simulink library "DAQ_lib_HallPositionTorque"  (R2014b)
settings: Solver=ode45  StartTime=0.0  StopTime=10.0  RelTol=1e-3
undefined symbols (not defined in the file): A_lpf_velocity, ANOMALY_INIT, B1_lpf_velocity, B2_lpf_velocity, Calibration, EnableFT, EncoderAngleLimits, EncoderFiltSys, EncoderThreshold, FTCalibration, GearOffsets, IMUAngleLimits, IMUCommand, IMUThreshold, IMUTorsoOffsets, m_XR17D15x, MAX_ANOMALY, MedullaCommand, MicrostrainFiltSys, MODBUS_TIMEOUT, ResetDAQ, ResetYaw, sample_time, standard, STREAMING_TIMEOUT, TareFT, TorsoCOMOffsets, Ts, TsCAN, TsKVH, UseMicrostrainRate
libraries: xpcethercatlib x207, simulink x53, canmsglib x21, speedgoatlib x13, slrtlib x5, speedgoatlib_IO601 x5, dspswit3 x2, dspmtrx3 x2, xpcseriallib x1, SpeedgoatModified x1
(part 1 of 7)
settings Model: Creator=rosshart  LastModifiedBy=rosshart

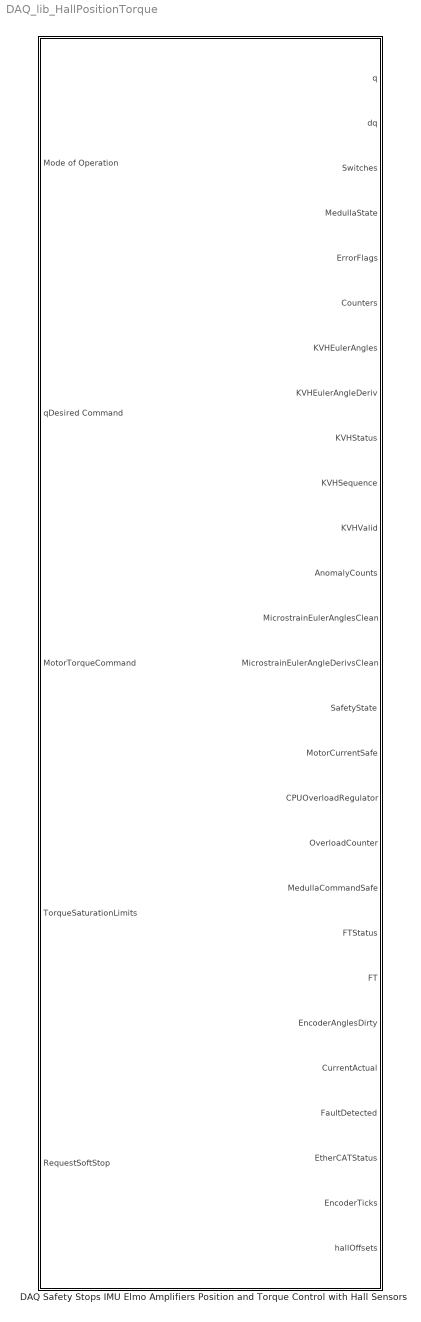
== system DAQ_lib_HallPositionTorque ==
  DAQ Safety Stops IMU Elmo Amplifiers Position and Torque Control with Hall Sensors : Subsystem  AncestorBlock=|
      | DAQ_lib/DAQ
      | Safety Stops
      | IMU
      | Elmo Amplifiers
      | Position and Torque Control with Hall Sensors

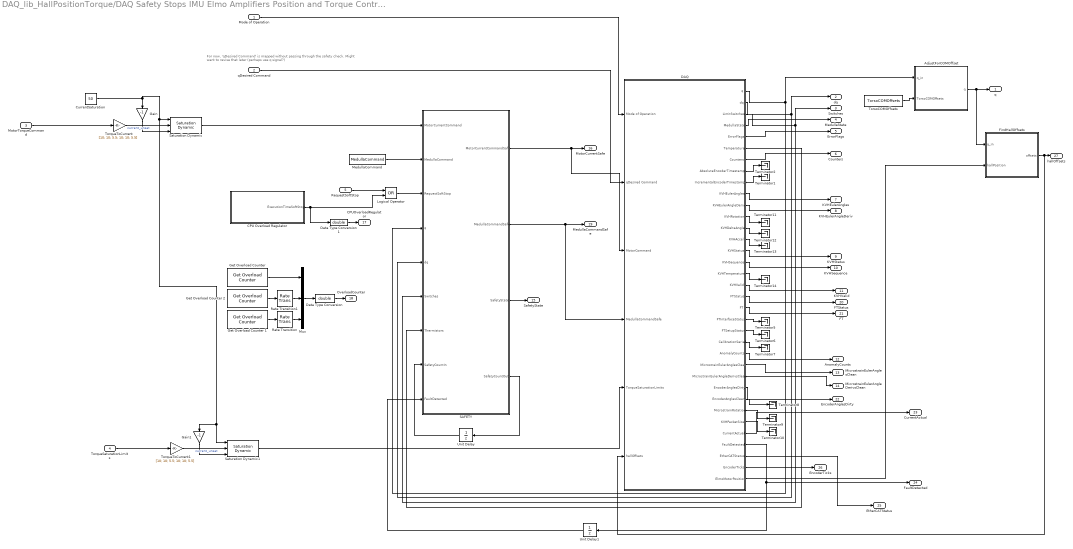
== system DAQ_lib_HallPositionTorque/DAQ Safety Stops IMU Elmo Amplifiers Position and Torque Control with Hall Sensors ==
  note: For now, 'qDesired Command' is mapped without passing through the safety check.
      | Might want to revise that later (perhaps use q signal?)
  Mode of Operation : Inport
  qDesired Command : Inport  Port=2
  MotorTorqueCommand : Inport  Port=3
  TorqueSaturationLimits : Inport  Port=4
  RequestSoftStop : Inport  Port=5
  AdjustForCOMOffset : MATLAB Function  TreatAsAtomicUnit=on
  CPU Overload Regulator : Subsystem
  CurrentSaturation : Constant  Value=50
  DAQ : Subsystem
  Data Type Conversion : DataTypeConversion  OutDataTypeStr=double
  Data Type Conversion1 : DataTypeConversion  OutDataTypeStr=double
  FindHallOffsets : MATLAB Function  TreatAsAtomicUnit=on
  Gain : Gain  Gain=-1
  Gain1 : Gain  Gain=-1
  "Get Overload Counter " : slrtlib/Target Management/Execution Parameters/Get Overload Counter   ts=Ts
  Get Overload Counter 1 : slrtlib/Target Management/Execution Parameters/Get Overload Counter   ts=TsMicrostrain
  Get Overload Counter 2 : slrtlib/Target Management/Execution Parameters/Get Overload Counter   ts=TsKVH
  Logical Operator : Logic  Operator=OR  OutDataTypeStr=boolean
  MedullaCommand : Constant  Value=MedullaCommand
  Mux : Mux  Inputs=3
  Rate Transition : RateTransition
  Rate Transition1 : RateTransition
  SAFETY : MATLAB Function  TreatAsAtomicUnit=on
  Saturation Dynamic : simulink/Discontinuities/Saturation Dynamic  OutMin=[]  OutMax=[]  OutDataTypeStr=Inherit: Same as second input  OutDataType=fixdt(1, 16)  OutScaling=2^-10  DoSatur=off
  Saturation Dynamic1 : simulink/Discontinuities/Saturation Dynamic  OutMin=[]  OutMax=[]  OutDataTypeStr=Inherit: Same as second input  OutDataType=fixdt(1, 16)  OutScaling=2^-10  DoSatur=off
  Terminator{1..2,5..14} (12 alike) : Terminator
  TorqueToCurrent : Gain  Gain=[10; 10; 5.5; 10; 10; 5.5]
  TorqueToCurrent1 : Gain  Gain=[10; 10; 5.5; 10; 10; 5.5]
  TorsoCOMOffsets : Constant  Value=TorsoCOMOffsets
  Unit Delay : UnitDelay  SampleTime=-1
  Unit Delay1 : UnitDelay  SampleTime=-1
  q : Outport
  dq : Outport  Port=2
  Switches : Outport  Port=3
  MedullaState : Outport  Port=4
  ErrorFlags : Outport  Port=5
  Counters : Outport  Port=6
  KVHEulerAngles : Outport  Port=7
  KVHEulerAngleDeriv : Outport  Port=8
  KVHStatus : Outport  Port=9
  KVHSequence : Outport  Port=10
  KVHValid : Outport  Port=11
  AnomalyCounts : Outport  Port=12
  MicrostrainEulerAnglesClean : Outport  Port=13
  MicrostrainEulerAngleDerivsClean : Outport  Port=14
  SafetyState : Outport  Port=15
  MotorCurrentSafe : Outport  Port=16
  CPUOverloadRegulator : Outport  Port=17
  OverloadCounter : Outport  Port=18
  MedullaCommandSafe : Outport  Port=19
  FTStatus : Outport  Port=20
  FT : Outport  Port=21
  EncoderAnglesDirty : Outport  Port=22
  CurrentActual : Outport  Port=23
  FaultDetected : Outport  Port=24
  EtherCATStatus : Outport  Port=25
  EncoderTicks : Outport  Port=26
  hallOffsets : Outport  Port=27
  wires:
  FindHallOffsets/1(offsets) -> hallOffsets/1, DAQ/6(hallOffsets)
  DAQ/35(ElmoMotorPosition) -> FindHallOffsets/2(hallPosition)
  TorqueSaturationLimits/1 -> TorqueToCurrent1/1
  TorqueToCurrent1/1 -> Saturation Dynamic1/2  "current_unsat"
  Gain1/1 -> Saturation Dynamic1/3
  Saturation Dynamic1/1 -> DAQ/5(TorqueSaturationLimits)
  DAQ/34(EncoderTicks) -> EncoderTicks/1
  DAQ/33(EtherCATStatus) -> EtherCATStatus/1
  MotorTorqueCommand/1 -> TorqueToCurrent/1
  DAQ/1(q) -> AdjustForCOMOffset/1(q_in), SAFETY/4(q)
  DAQ/2(dq) -> dq/1, SAFETY/5(dq)
  DAQ/3(LimitSwitches) -> Switches/1, SAFETY/6(Switches)
  SAFETY/3(SafetyState) -> SafetyState/1
  TorqueToCurrent/1 -> Saturation Dynamic/2  "current_unsat"
  DAQ/4(MedullaState) -> MedullaState/1
  DAQ/5(ErrorFlags) -> ErrorFlags/1
  Gain/1 -> Saturation Dynamic/3
  Saturation Dynamic/1 -> SAFETY/1(MotorCurrentCommand)
  SAFETY/2(MedullaCommandSafe) -> DAQ/4(MedullaCommandSafe), MedullaCommandSafe/1
  SAFETY/4(SafetyCountOut) -> Unit Delay/1
  Unit Delay/1 -> SAFETY/8(SafetyCountIn)
  DAQ/6(Temperature) -> SAFETY/7(Thermistors)
  DAQ/7(Counters) -> Counters/1
  AdjustForCOMOffset/1(q) -> q/1, FindHallOffsets/1(q_in)
  SAFETY/1(MotorCurrentCommandSafe) -> MotorCurrentSafe/1, DAQ/3(MotorCommand)
  DAQ/10(KVHEulerAngles) -> KVHEulerAngles/1
  DAQ/11(KVHEulerAngleDeriv) -> KVHEulerAngleDeriv/1
  DAQ/16(KVHSequence) -> KVHSequence/1
  DAQ/18(KVHValid) -> KVHValid/1
  DAQ/15(KVHStatus) -> KVHStatus/1
  DAQ/9(IncrementalEncoderTimestamps) -> Terminator1/1
  DAQ/24(AnomalyCounts) -> AnomalyCounts/1
  DAQ/8(AbsoluteEncoderTimestamps) -> Terminator2/1
  DAQ/25(MicrostrainEulerAnglesClean) -> MicrostrainEulerAnglesClean/1
  DAQ/26(MicrostrainEulerAngleDerivsClean) -> MicrostrainEulerAngleDerivsClean/1
  Logical Operator/1 -> SAFETY/3(RequestSoftStop)
  RequestSoftStop/1 -> Logical Operator/1
  CPU Overload Regulator/1(ExecutionTimeSoftStop) -> Logical Operator/2, Data Type Conversion1/1
  Data Type Conversion1/1 -> CPUOverloadRegulator/1
  MedullaCommand/1 -> SAFETY/2(MedullaCommand)
  CurrentSaturation/1 -> Gain/1, Saturation Dynamic/1, Saturation Dynamic1/1, Gain1/1
  TorsoCOMOffsets/1 -> AdjustForCOMOffset/2(TorsoCOMOffsets)
  DAQ/28(EncoderAnglesClean) -> Terminator8/1
  DAQ/29(MicrostrainRotation) -> Terminator9/1
  DAQ/30(KVHPacketSize) -> Terminator10/1
  DAQ/19(FTStatus) -> FTStatus/1
  DAQ/20(FT) -> FT/1
  DAQ/21(FTInterfaceStatus) -> Terminator5/1
  DAQ/23(CalibrationSerial) -> Terminator7/1
  DAQ/22(FTSetupStatus) -> Terminator6/1
  DAQ/14(KVHAccel) -> Terminator13/1
  DAQ/13(KVHDeltaAngle) -> Terminator12/1
  DAQ/12(KVHRotation) -> Terminator11/1
  DAQ/17(KVHTemperature) -> Terminator14/1
  "Get Overload Counter "/1 -> Mux/1
  Data Type Conversion/1 -> OverloadCounter/1
  Get Overload Counter 1/1 -> Rate Transition/1
  Mux/1 -> Data Type Conversion/1
  Rate Transition/1 -> Mux/3
  Get Overload Counter 2/1 -> Rate Transition1/1
  Rate Transition1/1 -> Mux/2
  DAQ/27(EncoderAnglesDirty) -> EncoderAnglesDirty/1
  DAQ/31(CurrentActual) -> CurrentActual/1
  DAQ/32(FaultDetected) -> Unit Delay1/1, FaultDetected/1
  Unit Delay1/1 -> SAFETY/9(FaultDetected)
  qDesired Command/1 -> DAQ/2(qDesired Command)
  Mode of Operation/1 -> DAQ/1(Mode of Operation)

== system DAQ_lib_HallPositionTorque/DAQ Safety Stops IMU Elmo Amplifiers Position and Torque Control with Hall Sensors/CPU Overload Regulator ==
  Bias : Bias  Bias=-1
  Compare To Constant : simulink/Logic and Bit Operations/Compare To Constant  relop=>=  const=Ts  OutDataTypeStr=boolean
  Compare To Constant1 : simulink/Logic and Bit Operations/Compare To Constant  relop=>=  const=Ts*10  OutDataTypeStr=boolean
  Compare To Zero : simulink/Logic and Bit Operations/Compare To Zero  relop===  OutDataTypeStr=boolean
  Reset CPU Overload Count : Subsystem  TreatAsAtomicUnit=on
  ResetExecutionDelaySteps : Constant  Value=50  SampleTime=Ts
  Resettable Delay : Delay  DelayLength=1  InitialConditionSource=Input port  ExternalReset=Level hold
      settings: InputPortMap=u0,r5,p4
  "Task Execution Time " : slrtlib/Target Management/Execution Parameters/Task Execution Time   ts=Ts
  ExecutionTimeSoftStop : Outport
  wires:
  Compare To Constant/1 -> Resettable Delay/2
  ResetExecutionDelaySteps/1 -> Resettable Delay/3
  "Task Execution Time "/1 -> Compare To Constant1/1, Compare To Constant/1
  Compare To Zero/1 -> Reset CPU Overload Count/Enable
  Compare To Constant1/1 -> ExecutionTimeSoftStop/1  "Request Soft Stop"
  Resettable Delay/1 -> Compare To Zero/1, Bias/1
  Bias/1 -> Resettable Delay/1

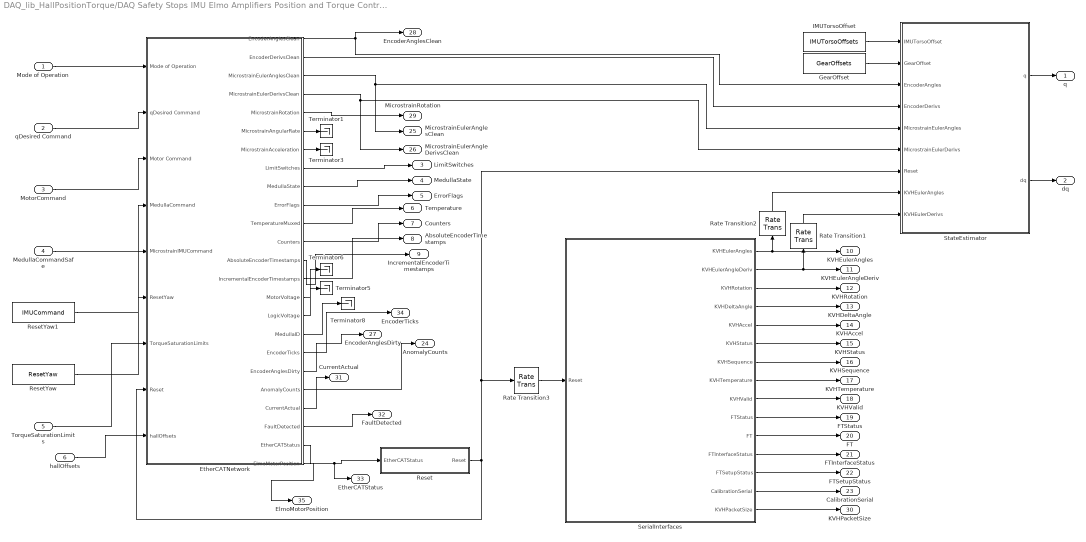
== system DAQ_lib_HallPositionTorque/DAQ Safety Stops IMU Elmo Amplifiers Position and Torque Control with Hall Sensors/DAQ ==
  Mode of Operation : Inport
  qDesired Command : Inport  Port=2
  MotorCommand : Inport  Port=3
  MedullaCommandSafe : Inport  Port=4
  TorqueSaturationLimits : Inport  Port=5
  hallOffsets : Inport  Port=6
  EtherCATNetwork : Subsystem
  GearOffset : Constant  Value=GearOffsets
  IMUTorsoOffset : Constant  Value=IMUTorsoOffsets
  Rate Transition1 : RateTransition  OutPortSampleTime=Ts
  Rate Transition2 : RateTransition  OutPortSampleTime=Ts
  Rate Transition3 : RateTransition  OutPortSampleTime=0.001
  Reset : Subsystem
  ResetYaw : Constant  Value=ResetYaw  OutDataTypeStr=boolean
  ResetYaw1 : Constant  Value=IMUCommand
  SerialInterfaces : Subsystem  TreatAsAtomicUnit=on  SystemSampleTime=TsKVH
  StateEstimator : Subsystem
  Terminator{1,3,5..6,8} (5 alike) : Terminator
  q : Outport
  dq : Outport  Port=2
  LimitSwitches : Outport  Port=3
  MedullaState : Outport  Port=4
  ErrorFlags : Outport  Port=5
  Temperature : Outport  Port=6
  Counters : Outport  Port=7
  AbsoluteEncoderTimestamps : Outport  Port=8
  IncrementalEncoderTimestamps : Outport  Port=9
  KVHEulerAngles : Outport  Port=10
  KVHEulerAngleDeriv : Outport  Port=11
  KVHRotation : Outport  Port=12
  KVHDeltaAngle : Outport  Port=13
  KVHAccel : Outport  Port=14
  KVHStatus : Outport  Port=15
  KVHSequence : Outport  Port=16
  KVHTemperature : Outport  Port=17
  KVHValid : Outport  Port=18
  FTStatus : Outport  Port=19
  FT : Outport  Port=20
  FTInterfaceStatus : Outport  Port=21
  FTSetupStatus : Outport  Port=22
  CalibrationSerial : Outport  Port=23
  AnomalyCounts : Outport  Port=24
  MicrostrainEulerAnglesClean : Outport  Port=25
  MicrostrainEulerAngleDerivsClean : Outport  Port=26
  EncoderAnglesDirty : Outport  Port=27
  EncoderAnglesClean : Outport  Port=28
  MicrostrainRotation : Outport  Port=29
  KVHPacketSize : Outport  Port=30
  CurrentActual : Outport  Port=31
  FaultDetected : Outport  Port=32
  EtherCATStatus : Outport  Port=33
  EncoderTicks : Outport  Port=34
  ElmoMotorPosition : Outport  Port=35
  wires:
  hallOffsets/1 -> EtherCATNetwork/9(hallOffsets)
  EtherCATNetwork/24(ElmoMotorPosition) -> ElmoMotorPosition/1
  TorqueSaturationLimits/1 -> EtherCATNetwork/7(TorqueSaturationLimits)
  ResetYaw/1 -> EtherCATNetwork/6(ResetYaw)
  Rate Transition3/1 -> SerialInterfaces/1(Reset)
  EtherCATNetwork/19(EncoderAnglesDirty) -> EncoderAnglesDirty/1
  SerialInterfaces/15(KVHPacketSize) -> KVHPacketSize/1
  EtherCATNetwork/6(MicrostrainAngularRate) -> Terminator1/1
  EtherCATNetwork/2(EncoderDerivsClean) -> StateEstimator/4(EncoderDerivs)
  Rate Transition1/1 -> StateEstimator/9(KVHEulerDerivs)
  EtherCATNetwork/10(ErrorFlags) -> ErrorFlags/1
  EtherCATNetwork/8(LimitSwitches) -> LimitSwitches/1
  EtherCATNetwork/5(MicrostrainRotation) -> MicrostrainRotation/1
  EtherCATNetwork/15(MotorVoltage) -> Terminator6/1
  EtherCATNetwork/14(IncrementalEncoderTimestamps) -> IncrementalEncoderTimestamps/1
  EtherCATNetwork/16(LogicVoltage) -> Terminator5/1
  EtherCATNetwork/17(MedullaID) -> Terminator8/1
  SerialInterfaces/3(KVHRotation) -> KVHRotation/1
  SerialInterfaces/1(KVHEulerAngles) -> KVHEulerAngles/1, Rate Transition2/1
  MotorCommand/1 -> EtherCATNetwork/3(Motor Command)
  SerialInterfaces/11(FT) -> FT/1
  StateEstimator/1(q) -> q/1
  IMUTorsoOffset/1 -> StateEstimator/1(IMUTorsoOffset)
  SerialInterfaces/13(FTSetupStatus) -> FTSetupStatus/1
  EtherCATNetwork/20(AnomalyCounts) -> AnomalyCounts/1
  EtherCATNetwork/12(Counters) -> Counters/1
  EtherCATNetwork/9(MedullaState) -> MedullaState/1
  StateEstimator/2(dq) -> dq/1
  EtherCATNetwork/13(AbsoluteEncoderTimestamps) -> AbsoluteEncoderTimestamps/1
  SerialInterfaces/10(FTStatus) -> FTStatus/1
  SerialInterfaces/12(FTInterfaceStatus) -> FTInterfaceStatus/1
  SerialInterfaces/2(KVHEulerAngleDeriv) -> KVHEulerAngleDeriv/1, Rate Transition1/1
  SerialInterfaces/8(KVHTemperature) -> KVHTemperature/1
  EtherCATNetwork/11(TemperatureMuxed) -> Temperature/1
  EtherCATNetwork/7(MicrostrainAcceleration) -> Terminator3/1
  EtherCATNetwork/18(EncoderTicks) -> EncoderTicks/1
  SerialInterfaces/14(CalibrationSerial) -> CalibrationSerial/1
  SerialInterfaces/5(KVHAccel) -> KVHAccel/1
  SerialInterfaces/7(KVHSequence) -> KVHSequence/1
  SerialInterfaces/9(KVHValid) -> KVHValid/1
  SerialInterfaces/6(KVHStatus) -> KVHStatus/1
  SerialInterfaces/4(KVHDeltaAngle) -> KVHDeltaAngle/1
  GearOffset/1 -> StateEstimator/2(GearOffset)
  EtherCATNetwork/3(MicrostrainEulerAnglesClean) -> MicrostrainEulerAnglesClean/1, StateEstimator/5(MicrostrainEulerAngles)
  EtherCATNetwork/4(MicrostrainEulerDerivsClean) -> StateEstimator/6(" MicrostrainEulerDerivs"), MicrostrainEulerAngleDerivsClean/1
  Reset/1(Reset) -> StateEstimator/7(Reset), Rate Transition3/1, EtherCATNetwork/8(Reset)
  Rate Transition2/1 -> StateEstimator/8(KVHEulerAngles)
  EtherCATNetwork/1(EncoderAnglesClean) -> EncoderAnglesClean/1, StateEstimator/3(EncoderAngles)
  MedullaCommandSafe/1 -> EtherCATNetwork/4(MedullaCommand)
  ResetYaw1/1 -> EtherCATNetwork/5(MicrostrainIMUCommand)
  EtherCATNetwork/21(CurrentActual) -> CurrentActual/1
  EtherCATNetwork/22(FaultDetected) -> FaultDetected/1
  qDesired Command/1 -> EtherCATNetwork/2(qDesired Command)
  EtherCATNetwork/23(EtherCATStatus) -> EtherCATStatus/1, Reset/1(EtherCATStatus)
  Mode of Operation/1 -> EtherCATNetwork/1(Mode of Operation)

== system DAQ_lib_HallPositionTorque/DAQ Safety Stops IMU Elmo Amplifiers Position and Torque Control with Hall Sensors/CPU Overload Regulator/Reset CPU Overload Count ==
  Enable : EnablePort
  Constant1 : Constant  Value=0
  Set Overload Counter 1 : slrtlib/Target Management/Execution Parameters/Set Overload Counter   ts=-1
  wires:
  Constant1/1 -> Set Overload Counter 1/1

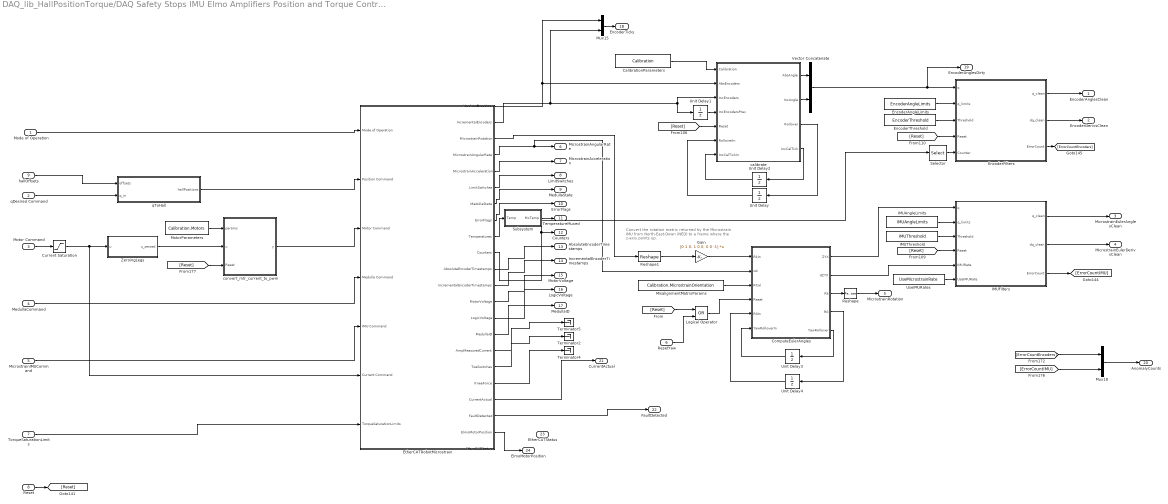
== system DAQ_lib_HallPositionTorque/DAQ Safety Stops IMU Elmo Amplifiers Position and Torque Control with Hall Sensors/DAQ/EtherCATNetwork ==
  note: Convert the rotation matrix returned by the
      | Microstrain IMU from North-East-Down
      | (NED) to a frame where the z-axis points up.
  Mode of Operation : Inport
  qDesired Command : Inport  Port=2
  Motor Command : Inport  Port=3
  MedullaCommand : Inport  Port=4
  MicrostrainIMUCommand : Inport  Port=5
  ResetYaw : Inport  Port=6
  TorqueSaturationLimits : Inport  Port=7
  Reset : Inport  Port=8
  hallOffsets : Inport  Port=9
  CalibrationParameters : Constant  Value=Calibration  OutDataTypeStr=Bus: RobotCalibrationBus
  ComputeEulerAngles : MATLAB Function  TreatAsAtomicUnit=on
  Current Saturation : Saturate  UpperLimit=50  LowerLimit=-50
  EncoderAngleLimits : Constant  Value=EncoderAngleLimits
  EncoderFilters : Subsystem  TreatAsAtomicUnit=on
  EncoderThreshold : Constant  Value=EncoderThreshold
  EtherCATRobotMicrostrain : Subsystem
  Gain : Gain  Gain=[0 1 0; 1 0 0; 0 0 -1]  Multiplication=Matrix(K*u)
  IMUAngleLimits : Constant  Value=IMUAngleLimits
  IMUFilters : Subsystem  TreatAsAtomicUnit=on
  IMUThreshold : Constant  Value=IMUThreshold
  Logical Operator : Logic  Operator=OR  OutDataTypeStr=boolean
  MisalignmentMatrixParams : Constant  Value=Calibration.MicrostrainOrientation
  MotorParameters : Constant  Value=Calibration.Motors
  Mux15 : Mux  Inputs=2
  Mux18 : Mux  Inputs=2
  Reshape : Reshape
  Reshape1 : Reshape  OutputDimensionality=Customize  OutputDimensions=[3,3]
  Selector : Selector  IndexMode=Zero-based  InputPortWidth=7  Indices=[0 1 3 4 0 1 3 4 2 5 0 1 3 4 2 5 6 6 6]
  Subsystem : Subsystem
  Terminator2 : Terminator
  Terminator4 : Terminator
  Terminator5 : Terminator
  Unit Delay : UnitDelay  InitialCondition=zeros(9,1)  SampleTime=-1
  Unit Delay1 : UnitDelay  SampleTime=-1
  Unit Delay2 : UnitDelay  InitialCondition=zeros(6,1)  SampleTime=-1
  Unit Delay3 : UnitDelay  InitialCondition=[0; 0]  SampleTime=-1
  Unit Delay4 : UnitDelay  InitialCondition=zeros(3,3)  SampleTime=-1
  UseIMURates : Constant  Value=UseMicrostrainRate
  Vector Concatenate : Concatenate
  ZeroingLegs : MATLAB Function  TreatAsAtomicUnit=on
  calibrate : MATLAB Function  TreatAsAtomicUnit=on
  convert_mtr_current_to_pwm : MATLAB Function  TreatAsAtomicUnit=on
  qToHall : MATLAB Function  TreatAsAtomicUnit=on
  EncoderAnglesClean : Outport
  EncoderDerivsClean : Outport  Port=2
  MicrostrainEulerAnglesClean : Outport  Port=3
  MicrostrainEulerDerivsClean : Outport  Port=4
  MicrostrainRotation : Outport  Port=5
  MicrostrainAngularRate : Outport  Port=6
  MicrostrainAcceleration : Outport  Port=7
  LimitSwitches : Outport  Port=8
  MedullaState : Outport  Port=9
  ErrorFlags : Outport  Port=10
  TemperatureMuxed : Outport  Port=11
  Counters : Outport  Port=12
  AbsoluteEncoderTimestamps : Outport  Port=13
  IncrementalEncoderTimestamps : Outport  Port=14
  MotorVoltage : Outport  Port=15
  LogicVoltage : Outport  Port=16
  MedullaID : Outport  Port=17
  EncoderTicks : Outport  Port=18
  EncoderAnglesDirty : Outport  Port=19
  AnomalyCounts : Outport  Port=20
  CurrentActual : Outport  Port=21
  FaultDetected : Outport  Port=22
  EtherCATStatus : Outport  Port=23
  ElmoMotorPosition : Outport  Port=24
  wires:
  hallOffsets/1 -> qToHall/1(offsets)
  EtherCATRobotMicrostrain/21(ElmoMotorPosition) -> ElmoMotorPosition/1
  ? -> EtherCATStatus/1
  TorqueSaturationLimits/1 -> EtherCATRobotMicrostrain/7(TorqueSaturationLimits)
  EtherCATRobotMicrostrain/17(ToeSwitches) -> Terminator2/1
  EtherCATRobotMicrostrain/16(AmpMeasuredCurrent) -> Terminator5/1
  MicrostrainIMUCommand/1 -> EtherCATRobotMicrostrain/5(IMU Command)
  MedullaCommand/1 -> EtherCATRobotMicrostrain/4(Medulla Command)
  CalibrationParameters/1 -> calibrate/1(Calibration)
  calibrate/3(Rollover) -> Unit Delay/1
  Unit Delay/1 -> calibrate/6(RolloverIn)
  [Reset] -> calibrate/5(Reset)
  Unit Delay1/1 -> calibrate/4(IncEncodersPrev)
  Unit Delay2/1 -> calibrate/7(IncCalTickIn)
  calibrate/4(IncCalTick) -> Unit Delay2/1
  [Reset] -> convert_mtr_current_to_pwm/3(Reset)
  Motor Command/1 -> Current Saturation/1
  MotorParameters/1 -> convert_mtr_current_to_pwm/1(params)
  Current Saturation/1 -> EtherCATRobotMicrostrain/6(Current Command), ZeroingLegs/1(u)
  convert_mtr_current_to_pwm/1(y) -> EtherCATRobotMicrostrain/3(Motor Command)
  Mux15/1 -> EncoderTicks/1
  EtherCATRobotMicrostrain/18(KneeForce) -> Terminator4/1
  EtherCATRobotMicrostrain/7(MedullaState) -> MedullaState/1
  Subsystem/1(MxTemp) -> TemperatureMuxed/1
  EtherCATRobotMicrostrain/9(Temperatures) -> Subsystem/1(Temp)
  EtherCATRobotMicrostrain/8(ErrorFlags) -> ErrorFlags/1
  EtherCATRobotMicrostrain/6(LimitSwitches) -> LimitSwitches/1
  EtherCATRobotMicrostrain/13(MotorVoltage) -> MotorVoltage/1
  EtherCATRobotMicrostrain/14(LogicVoltage) -> LogicVoltage/1
  EtherCATRobotMicrostrain/5(MicrostrainAcceleration) -> MicrostrainAcceleration/1
  EtherCATRobotMicrostrain/11(AbsoluteEncoderTimestamps) -> AbsoluteEncoderTimestamps/1
  EtherCATRobotMicrostrain/12(IncrementalEncoderTimestamps) -> IncrementalEncoderTimestamps/1
  EtherCATRobotMicrostrain/15(MedullaID) -> MedullaID/1
  EtherCATRobotMicrostrain/1(AbsoluteEncoders) -> Mux15/1, calibrate/2(AbsEncoders)
  EtherCATRobotMicrostrain/2(IncrementalEncoders) -> Mux15/2, calibrate/3(IncEncoders), Unit Delay1/1
  ComputeEulerAngles/1(ZYX) -> IMUFilters/1(q)
  [Reset] -> IMUFilters/4(Reset)
  IMUFilters/3(ErrorCount) -> [ErrorCountIMU]
  IMUThreshold/1 -> IMUFilters/3(Threshold)
  EtherCATRobotMicrostrain/10(Counters) -> Counters/1, Selector/1
  IMUAngleLimits/1 -> IMUFilters/2(q_limits)
  Selector/1 -> EncoderFilters/5(Counter)
  UseIMURates/1 -> IMUFilters/6(UseIMURate)
  EncoderFilters/3(ErrorCount) -> [ErrorCountEncoders]
  IMUFilters/2(dq_clean) -> MicrostrainEulerDerivsClean/1
  [Reset] -> EncoderFilters/4(Reset)
  EncoderAngleLimits/1 -> EncoderFilters/2(q_limits)
  EncoderFilters/1(q_clean) -> EncoderAnglesClean/1
  IMUFilters/1(q_clean) -> MicrostrainEulerAnglesClean/1
  EncoderFilters/2(dq_clean) -> EncoderDerivsClean/1
  EncoderThreshold/1 -> EncoderFilters/3(Threshold)
  calibrate/1(AbsAngle) -> Vector Concatenate/1
  calibrate/2(IncAngle) -> Vector Concatenate/2
  Vector Concatenate/1 -> EncoderAnglesDirty/1, EncoderFilters/1(q)
  ComputeEulerAngles/2(dZYX) -> IMUFilters/5(IMURate)
  Mux18/1 -> AnomalyCounts/1
  [ErrorCountEncoders] -> Mux18/1
  [ErrorCountIMU] -> Mux18/2
  MisalignmentMatrixParams/1 -> ComputeEulerAngles/3(RCal)
  Unit Delay4/1 -> ComputeEulerAngles/5(R0In)
  ComputeEulerAngles/4(R0) -> Unit Delay4/1
  ComputeEulerAngles/3(Rk) -> Reshape/1
  [Reset] -> Logical Operator/1
  Reshape/1 -> MicrostrainRotation/1
  EtherCATRobotMicrostrain/3(MicrostrainRotation) -> Reshape1/1
  EtherCATRobotMicrostrain/4(MicrostrainAngularRate) -> MicrostrainAngularRate/1, ComputeEulerAngles/2(wk)
  ComputeEulerAngles/5(YawRollover) -> Unit Delay3/1
  Unit Delay3/1 -> ComputeEulerAngles/6(YawRolloverIn)
  ResetYaw/1 -> Logical Operator/2
  Logical Operator/1 -> ComputeEulerAngles/4(Reset)
  Reshape1/1 -> Gain/1
  Gain/1 -> ComputeEulerAngles/1(RkIn)
  Reset/1 -> [Reset]
  EtherCATRobotMicrostrain/19(CurrentActual) -> CurrentActual/1
  EtherCATRobotMicrostrain/20(FaultDetected) -> FaultDetected/1
  ZeroingLegs/1(u_zeroed) -> convert_mtr_current_to_pwm/2(u)
  qDesired Command/1 -> qToHall/2(q_in)
  Mode of Operation/1 -> EtherCATRobotMicrostrain/1(Mode of Operation)
  qToHall/1(hallPositions) -> EtherCATRobotMicrostrain/2(Position Command)

== system DAQ_lib_HallPositionTorque/DAQ Safety Stops IMU Elmo Amplifiers Position and Torque Control with Hall Sensors/DAQ/Reset ==
  note: EtherCATStatus is a vector of six elements:
      | [ErrVal MasterState DCErrVal MasterToNetworkClkDiff
      | DCInitState NetworkToSlaveClkDiff]
      | Here we just check that MasterState==8 (Operational state),
      | the DC is started, and that there is no DC error.
  EtherCATStatus : Inport
  Compare To Constant : simulink/Logic and Bit Operations/Compare To Constant  relop=<=  const=12.0  OutDataTypeStr=boolean
  Compare To Constant1 : simulink/Logic and Bit Operations/Compare To Constant  relop=~=  const=8  OutDataTypeStr=boolean
  Compare To Constant2 : simulink/Logic and Bit Operations/Compare To Constant  relop=>  const=0  OutDataTypeStr=boolean
  Digital Clock : DigitalClock  SampleTime=Ts
  Logical Operator : Logic  Operator=OR  Inputs=3  OutDataTypeStr=boolean
  Logical Operator1 : Logic  Operator=OR  OutDataTypeStr=boolean
  Logical Operator2 : Logic  OutDataTypeStr=boolean
  ResetDAQ1 : Constant  Value=ResetDAQ  OutDataTypeStr=boolean
  Selector : Selector  IndexMode=Zero-based  InputPortWidth=6
  Selector1 : Selector  IndexMode=Zero-based  InputPortWidth=6  Indices=2
  Unit Delay : UnitDelay  InitialCondition=1  SampleTime=-1
  Reset : Outport
  wires:
  Selector/1 -> Compare To Constant1/1
  EtherCATStatus/1 -> Selector/1, Selector1/1
  Compare To Constant1/1 -> Logical Operator/2
  Digital Clock/1 -> Compare To Constant/1
  Compare To Constant/1 -> Logical Operator/1
  Selector1/1 -> Compare To Constant2/1
  Compare To Constant2/1 -> Logical Operator/3
  ResetDAQ1/1 -> Logical Operator1/1
  Logical Operator1/1 -> Reset/1
  Logical Operator/1 -> Logical Operator2/1
  Unit Delay/1 -> Logical Operator2/2, Logical Operator1/2
  Logical Operator2/1 -> Unit Delay/1

== system DAQ_lib_HallPositionTorque/DAQ Safety Stops IMU Elmo Amplifiers Position and Torque Control with Hall Sensors/DAQ/SerialInterfaces ==
  Reset : Inport
  EnableFT : Constant  Value=EnableFT  OutDataTypeStr=boolean
  FTCAN : Subsystem  Commented=on
  FTInterface : Subsystem  Commented=on
  KVH : Subsystem
  ResetYaw : Constant  Value=ResetYaw  OutDataTypeStr=boolean
  TareFT : Constant  Value=TareFT  OutDataTypeStr=boolean
  KVHEulerAngles : Outport
  KVHEulerAngleDeriv : Outport  Port=2
  KVHRotation : Outport  Port=3
  KVHDeltaAngle : Outport  Port=4
  KVHAccel : Outport  Port=5
  KVHStatus : Outport  Port=6
  KVHSequence : Outport  Port=7
  KVHTemperature : Outport  Port=8
  KVHValid : Outport  Port=9
  FTStatus : Outport  Port=10
  FT : Outport  Port=11
  FTInterfaceStatus : Outport  Port=12
  FTSetupStatus : Outport  Port=13
  CalibrationSerial : Outport  Port=14
  KVHPacketSize : Outport  Port=15
  wires:
  KVH/4(DeltaAngle) -> KVHDeltaAngle/1
  KVH/5(Accel) -> KVHAccel/1
  KVH/7(Sequence) -> KVHSequence/1
  KVH/6(Status) -> KVHStatus/1
  KVH/8(Temperature) -> KVHTemperature/1
  KVH/9(Valid) -> KVHValid/1
  ResetYaw/1 -> KVH/1(ResetYaw)
  KVH/1(EulerAngles) -> KVHEulerAngles/1
  KVH/2(EulerAngleDerivatives) -> KVHEulerAngleDeriv/1
  FTInterface/4(FTSetupStatus) -> ?
  FTInterface/1(FTStatus) -> ?
  FTInterface/5(CalibrationSerial) -> CalibrationSerial/1
  FTInterface/3(FTInterfaceStatus) -> ?
  TareFT/1 -> FTCAN/1(ZeroFT), FTInterface/1(Tare)
  Reset/1 -> FTInterface/2(Reset), KVH/2(Reset)
  FTInterface/2(FT) -> ?
  KVH/3(Rk) -> KVHRotation/1
  EnableFT/1 -> FTInterface/Enable
  KVH/10(PacketSize) -> KVHPacketSize/1
  FTCAN/1(PortStatus) -> FTInterfaceStatus/1
  FTCAN/2(Timeout) -> FTSetupStatus/1
  FTCAN/3(FTStatus) -> FTStatus/1
  FTCAN/4(FT) -> FT/1

== system DAQ_lib_HallPositionTorque/DAQ Safety Stops IMU Elmo Amplifiers Position and Torque Control with Hall Sensors/DAQ/StateEstimator ==
  IMUTorsoOffset : Inport
  GearOffset : Inport  Port=2
  EncoderAngles : Inport  Port=3
  EncoderDerivs : Inport  Port=4
  MicrostrainEulerAngles : Inport  Port=5
  " MicrostrainEulerDerivs" : Inport  Port=6
  Reset : Inport  Port=7
  KVHEulerAngles : Inport  Port=8
  KVHEulerDerivs : Inport  Port=9
  GeneralizedCoordinates : MATLAB Function  TreatAsAtomicUnit=on
  Switch : Switch  Criteria=u2 > Threshold
  Switch1 : Switch  Criteria=u2 > Threshold
  UseIMU : Constant
  UseKVH : Constant
  UseMotorIncEncoders : Constant  Value=0
  q : Outport
  dq : Outport  Port=2
  wires:
  UseIMU/1 -> GeneralizedCoordinates/6(UseIMU)
  GearOffset/1 -> GeneralizedCoordinates/8(GearOffset)
  UseMotorIncEncoders/1 -> GeneralizedCoordinates/5(UseMotorIncEncoders)
  IMUTorsoOffset/1 -> GeneralizedCoordinates/7(IMUTorsoOffset)
  GeneralizedCoordinates/2(dq_clean) -> dq/1
  GeneralizedCoordinates/1(q_clean) -> q/1
  Reset/1 -> GeneralizedCoordinates/9(Reset)
  EncoderAngles/1 -> GeneralizedCoordinates/1(EncoderAngles)
  EncoderDerivs/1 -> GeneralizedCoordinates/2(EncoderVelocities)
  KVHEulerAngles/1 -> Switch/1
  MicrostrainEulerAngles/1 -> Switch/3
  Switch/1 -> GeneralizedCoordinates/3(IMUAngles)
  UseKVH/1 -> Switch1/2, Switch/2
  KVHEulerDerivs/1 -> Switch1/1
  " MicrostrainEulerDerivs"/1 -> Switch1/3
  Switch1/1 -> GeneralizedCoordinates/4(IMUVelocities)

== system DAQ_lib_HallPositionTorque/DAQ Safety Stops IMU Elmo Amplifiers Position and Torque Control with Hall Sensors/DAQ/EtherCATNetwork/EncoderFilters ==
  q : Inport  Partition=on  PartitionDimension=1  PartitionWidth=1
  q_limits : Inport  Port=2  Partition=on  PartitionDimension=1  PartitionWidth=1
  Threshold : Inport  Port=3  Partition=on  PartitionDimension=1  PartitionWidth=1
  Reset : Inport  Port=4  Partition=off
  Counter : Inport  Port=5  Partition=on  PartitionDimension=1  PartitionWidth=1
  CheckAndFilterEncoder : Subsystem
  For Each : ForEach  DisableCoverage=on  IndexMode=One-based
  q_clean : Outport  ConcatenationDimension=1
  dq_clean : Outport  Port=2  ConcatenationDimension=1
  ErrorCount : Outport  Port=3  ConcatenationDimension=1
  wires:
  Counter/1 -> CheckAndFilterEncoder/5(Counter)
  Reset/1 -> CheckAndFilterEncoder/4(Reset)
  CheckAndFilterEncoder/2(dq_clean) -> dq_clean/1
  q_limits/1 -> CheckAndFilterEncoder/2(q_limits)
  CheckAndFilterEncoder/3(ErrorCount) -> ErrorCount/1
  CheckAndFilterEncoder/1(q_clean) -> q_clean/1
  Threshold/1 -> CheckAndFilterEncoder/3(Threshold)
  q/1 -> CheckAndFilterEncoder/1(q_daq)
